simulink model "hvac_1zone_v3"  (R2021a)
settings: Solver=FixedStepDiscrete  StartTime=0.0  StopTime=Inf  FixedStep=60  RelTol=1e-3  EnableMultiTasking=on
values from neighbouring files (symbols this model uses):
  Ts2 = 600    [main_1zone.m]
undefined symbols (not defined in the file or in its folder): beta, ci, den, high, low, num, params1, rl, Ts
libraries: dspmathops x2, rllib x1
settings Model: Creator=User  LastModifiedBy=Richi
settings SolverCC: AlgebraicLoopSolver=TrustRegion
settings DataIOCC: LimitDataPoints=on  SaveFormat=Array  SignalLoggingSaveFormat=ModelDataLogs  SaveOutput=off  SaveTime=off
settings OptimizationCC: LifeSpan=inf
settings DebuggingCC: AlgebraicLoopMsg=none  ArtificialAlgebraicLoopMsg=none  SignalResolutionControl=None  InheritedTsInSrcMsg=none  MultiTaskDSMMsg=none  MultiTaskCondExecSysMsg=none  MultiTaskRateTransMsg=warning  TasksWithSamePriorityMsg=none  SigSpecEnsureSampleTimeMsg=none  IntegerOverflowMsg=none  Int32ToFloatConvMsg=none  ParameterPrecisionLossMsg=none  ParameterTunabilityLossMsg=none  UnconnectedInputMsg=none  UnconnectedOutputMsg=none  UnconnectedLineMsg=none  BusObjectLabelMismatch=none  RootOutportRequireBusObject=none  AllowSymbolicDim=off  UnknownTsInhSupMsg=none  ModelReferenceDataLoggingMessage=none  OperatingPointInterfaceChecksumMismatchMsg=none  SFUnusedDataAndEventsDiag=none  SFUnexpectedBacktrackingDiag=none  SFInvalidInputDataAccessInChartInitDiag=none  SFNoUnconditionalDefaultTransitionDiag=none  SFTransitionOutsideNaturalParentDiag=none  SFUnreachableExecutionPathDiag=none  SFUndirectedBroadcastEventsDiag=none  SFTransitionActionBeforeConditionDiag=none  SFTemporalDelaySmallerThanSampleTimeDiag=none  SFSelfTransitionDiag=none  SFExecutionAtInitializationDiag=none  SFMachineParentedDataDiag=none  IntegerSaturationMsg=none  ArithmeticOperatorsInVariantConditions=warning
settings HardwareCC: ProdBitPerPointer=32  ProdBitPerSizeT=32  ProdBitPerPtrDiffT=32  ProdLargestAtomicFloat=None  ProdIntDivRoundTo=Undefined  ProdEndianess=Unspecified  ProdWordSize=32  ProdHWDeviceType=32-bit Generic
settings ModelReferenceCC: PropagateSignalLabelsOutOfModel=off
settings SFSimCC: SimUseLocalCustomCode=off  CustomCodeUndefinedFunction=UseInterfaceOnly  SimTargetLang=C++
settings RTWCC: RTWUseLocalCustomCode=off
settings CodeAppCC: StateflowObjectComments=on
settings GRTTargetCC: TargetLangStandard=C89/C90 (ANSI)
settings ConfigComp: CovMetricSettings=dw  CovSaveCumulativeToWorkspaceVar=on  CovSaveSingleToWorkspaceVar=on  CovExternalEMLEnable=off

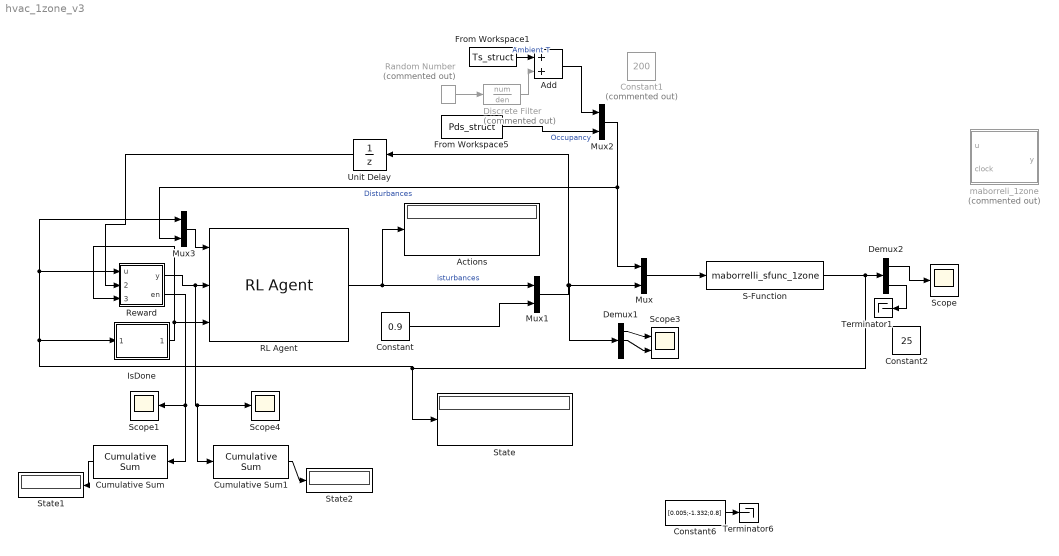
== system hvac_1zone_v3 ==
  " Reward" : MATLAB Function  TreatAsAtomicUnit=on  SystemSampleTime=Ts2
  Actions : Display
  Add : Sum
  Constant : Constant  Value=0.9
  Constant1 : Constant  Commented=on  Value=200
  Constant2 : Constant  Value=25
  Constant6 : Constant  Value=[0.005;-1.332;0.8]
  Cumulative Sum : dspmathops/Cumulative Sum  dim=Channels (running sum)  InputProcessing=Columns as channels (frame based)  reset_popup=None  roundingMode=Floor  overflowMode=off  outputDataTypeStr=Inherit: Same as accumulator  outputMin=[]  outputMax=[]  outputLastDataTypeStr=Inherit: Same as accumulator
  Cumulative Sum1 : dspmathops/Cumulative Sum  dim=Channels (running sum)  InputProcessing=Columns as channels (frame based)  reset_popup=None  roundingMode=Floor  overflowMode=off  outputDataTypeStr=Inherit: Same as accumulator  outputMin=[]  outputMax=[]  outputLastDataTypeStr=Inherit: Same as accumulator
  Demux1 : Demux  Outputs=3
  Demux2 : Demux  Outputs=2
  Discrete Filter : DiscreteFilter  Commented=on  Numerator=num  Denominator=den  SampleTime=5400
  From Workspace1 : FromWorkspace  VariableName=Ts_struct  OutDataTypeStr=double  SampleTime=Ts
  From Workspace5 : FromWorkspace  VariableName=Pds_struct  OutDataTypeStr=double  SampleTime=Ts
  IsDone : MATLAB Function  TreatAsAtomicUnit=on  SystemSampleTime=Ts2
  Mux{,1..3} (4 alike) : Mux  Inputs=2
  RL Agent : rllib/RL Agent  Agent=rl.util.PolicyInstance.get('hvac_1zone_v3/RL Agent')  ExternalActionAsInput=off  ProvideCumRwd=off  TreatAsDirectFeedthrough=on
  Random Number : RandomNumber  Commented=on  Variance=0.5  SampleTime=1800
  S-Function : S-Function  FunctionName=maborrelli_sfunc_1zone  Parameters=ci,params1,60  SFunctionDeploymentMode=off  EnableBusSupport=off
  Scope : Scope
  Scope1 : Scope
  Scope3 : Scope  NumInputPorts=2
  Scope4 : Scope
  State : Display
  State1 : Display
  State2 : Display
  Terminator1 : Terminator
  Terminator6 : Terminator
  Unit Delay : UnitDelay  SampleTime=Ts2  HasFrameUpgradeWarning=on
  maborreli_1zone : MATLAB Function  Commented=on  TreatAsAtomicUnit=on  SystemSampleTime=Ts
  wires:
  Mux2/1 -> Mux3/2, Mux/1  "Disturbances"
  From Workspace5/1 -> Mux2/2  "Occupancy"
  Mux/1 -> S-Function/1
  Constant6/1 -> Terminator6/1
  Discrete Filter/1 -> Add/2
  Random Number/1 -> Discrete Filter/1
  IsDone/1(value) -> " Reward"/3(isDone), RL Agent/3
  Demux1/2 -> Scope3/2
  Demux1/1 -> Scope3/1
  Demux2/1 -> Scope/1
  Demux2/2 -> Terminator1/1
  S-Function/1 -> Mux3/1, " Reward"/1(u), IsDone/1(states), State/1, Demux2/1
  RL Agent/1 -> Actions/1, Mux1/1  "isturbances"
  Unit Delay/1 -> " Reward"/2(actions)
  From Workspace1/1 -> Add/1  "Ambient T"
  Mux3/1 -> RL Agent/1
  Add/1 -> Mux2/1
  ? -> maborreli_1zone/2(clock)
  Mux1/1 -> Demux1/1, Mux/2, Unit Delay/1
  Constant/1 -> Mux1/2
  " Reward"/2(en) -> Cumulative Sum/1, Scope1/1
  Cumulative Sum/1 -> State1/1
  Cumulative Sum1/1 -> State2/1
  " Reward"/1(y) -> Cumulative Sum1/1, Scope4/1, RL Agent/2

== matlab function hvac_1zone_v3/IsDone ==
  data: states input; value output
function value = fcn(states)
 low = -20;
 max = 55;
 value = 0; 
 %disp(length(block.InputPort(1).Data))
 for i=1:length(states)
     %disp(i)
     if i == 3
         break
     end
     aux = states(i);
     %disp(aux)
     if (aux < low || aux > max) 
        %disp(abs(aux - low))
        value = 1;
        break
     end
     %disp('if3')
 end

== matlab function hvac_1zone_v3/ Reward ==
  data: u input; y output; actions input; isDone input; low parameter; high parameter; beta parameter; en output
function [y, en] = reward(u, actions, isDone, low, high, beta)
 ms = actions(1);
 Dt = actions(2);
 %Añadir energía:
 e = ((-1012/4)*ms*Dt+ 65*(ms)^2)/1000;
 reward = -beta* e; 
 en = e;
 %disp('reward por energia')
 %disp(reward)
 %disp(length(block.InputPort(1).Data))
 for i=1:1
     aux = u(i);
     %disp('estado')
     %disp(aux)
     if (aux < low || aux > high)
        reward = reward - 0.4*(min(abs(aux - low), abs(aux - high))+ (min( abs(aux - low), abs(aux - high)))^2);
        %disp('reward por estado')
        %disp(-min( abs(aux - low), abs(aux - high)))
     end
     %disp('if1')
     %if (aux >= low && aux <= high)
     %    reward = reward + 1;
     %end

 end
 if isDone
     reward = -2000;
 end
y = reward;

== matlab function hvac_1zone_v3/maborreli_1zone ==
  data: u input; y output; params1 parameter; ci parameter; Ts parameter; states data_store_memory; clock input
function y = fcn(u,params1, ci, Ts, clock)
ST = Ts;
params = params1;
global states;
dT = [0;0];
delta=u(5);
if clock == 0
    dT = ci;
else
    x = states;
    dT(1)=x(1)+(ST*u(3)*params.cp*((delta*x(1)+(1-delta)*u(1)+u(4))-x(1))+ ST*(x(2)-x(1))/params.R+...
        ST*(u(1)-x(1))/params.Roa+ST*u(2))/params.C1;
    dT(2)=x(2)+ST*(x(1)-x(2))/params.R/params.C2;
end
states = dT;
y = dT;
